simulink model "MDL_Tlepkie"  (R2023a)
settings: Solver=ode4  StartTime=0.0  StopTime=end_time  FixedStep=dt  MaxStep=0.001  RelTol=1e-3
values from neighbouring files (symbols this model uses):
  dt = 0.001    [anim_sim_script.m]
  IC = [x_ic, theta_ic, D_x_ic, D_theta_ic]'    [anim_sim_script.m]
settings Model: Creator=Adam  LastModifiedBy=Adam
settings SolverCC: AlgebraicLoopSolver=TrustRegion
settings DataIOCC: SaveOutput=off  SignalLogging=off  DSMLogging=off
settings DebuggingCC: AlgebraicLoopMsg=none  UnconnectedInputMsg=warning  UnconnectedOutputMsg=warning  UnconnectedLineMsg=warning
settings ModelReferenceCC: EnableRefExpFcnMdlSchedulingChecks=on
settings RTWCC: DLArmComputeVersion=19.05

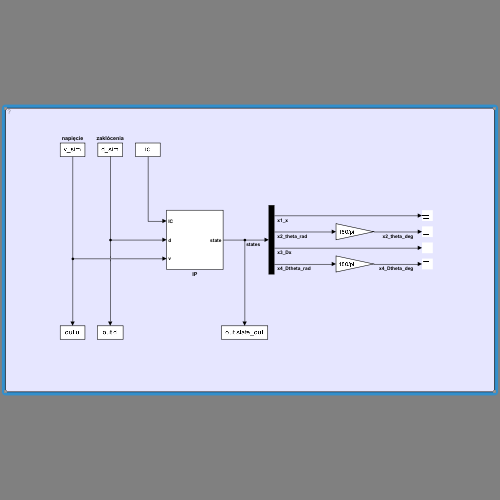
[thumbnail: Simulink's stored preview of the top-level diagram]
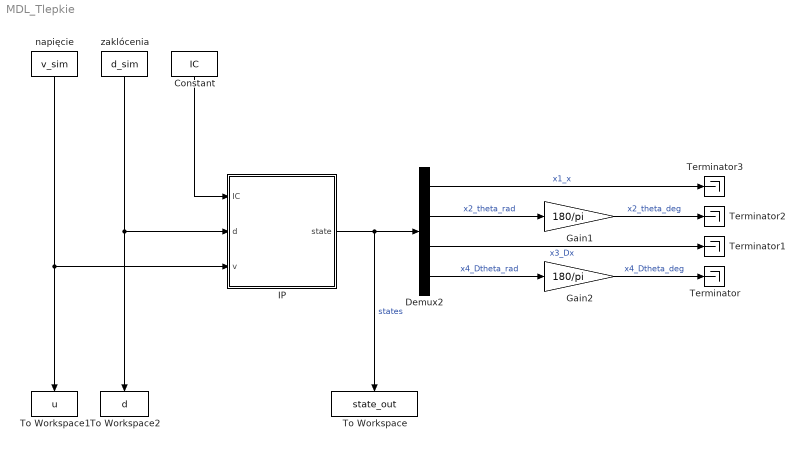
== system MDL_Tlepkie ==
  Constant : Constant  Value=IC
  Demux2 : Demux
  Gain1 : Gain  Gain=180/pi
  Gain2 : Gain  Gain=180/pi
  IP : Subsystem
  Terminator{,1..3} (4 alike) : Terminator
  To Workspace : ToWorkspace  VariableName=state_out  SampleTime=-1
  To Workspace1 : ToWorkspace  VariableName=u  SampleTime=-1
  To Workspace2 : ToWorkspace  VariableName=d  SampleTime=-1
  napięcie : FromWorkspace  VariableName=v_sim  SampleTime=dt
  zaklócenia : FromWorkspace  VariableName=d_sim  SampleTime=dt
  wires:
  Gain2/1 -> Terminator/1  "x4_Dtheta_deg"
  Demux2/4 -> Gain2/1  "x4_Dtheta_rad"
  Demux2/3 -> Terminator1/1  "x3_Dx"
  Demux2/2 -> Gain1/1  "x2_theta_rad"
  Demux2/1 -> Terminator3/1  "x1_x"
  Gain1/1 -> Terminator2/1  "x2_theta_deg"
  IP/1(state) -> Demux2/1, To Workspace/1  "states"
  napięcie/1 -> IP/3(v), To Workspace1/1
  zaklócenia/1 -> IP/2(d), To Workspace2/1
  Constant/1 -> IP/1(IC)

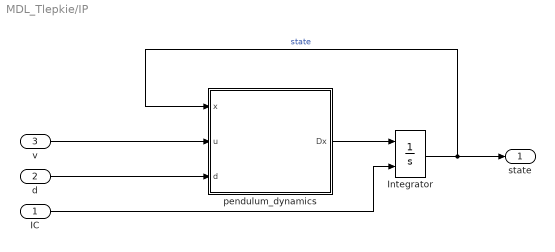
== system MDL_Tlepkie/IP ==
  IC : Inport
  d : Inport  Port=2
  v : Inport  Port=3
  Integrator : Integrator  InitialConditionSource=external
  pendulum_dynamics : MATLAB Function  TreatAsAtomicUnit=on
  state : Outport
  wires:
  Integrator/1 -> state/1, pendulum_dynamics/1(x)  "state"
  v/1 -> pendulum_dynamics/2(u)
  pendulum_dynamics/1(Dx) -> Integrator/1
  IC/1 -> Integrator/2
  d/1 -> pendulum_dynamics/3(d)

== matlab function MDL_Tlepkie/IP/pendulum_dynamics ==
  data: x input; u input; d input; Dx output; params_lepkie parameter
function Dx = dynamika_wahadla(x, u, d, params_lepkie)
% x : stan
% u : input - napięcie
%
% params scope: "parameters"
%

% State, function input: x = [x Dx theta Dtheta]'
x1 = x(1);
x2 = x(2); 
x3 = x(3);
x4 = x(4);

params_lepkie = num2cell(params_lepkie);
[M, mc, mp, Lp, Lc, g, b, gamma, mr, Mt, L, Jcm, Jt, alpha, beta] = params_lepkie{:};

% Equations for pendulum dynamics
Ff = b*x3;
Fi = alpha*u - beta*x3;
A = d*cos(x2) - Ff + L*mr*x4^2*sin(x2) + Fi;
B = d*Lc + L*g*mr*sin(x2) - gamma*x4;
DEN = Jt*Mt - (L*mr*cos(x2))^2;

ddt_x1 = x3;
ddt_x2 = x4;
ddt_x3 = (Jt*A - L*mr*cos(x2)*B) / DEN;
ddt_x4 = (Mt*B - L*mr*cos(x2)*A) / DEN;

% output
Dx = [ddt_x1 ddt_x2 ddt_x3 ddt_x4]';

end
